simulink model "TrailerSoftware"  (R2019b)
settings: Solver=FixedStepDiscrete  StartTime=0.0  StopTime=inf  FixedStep=update  RelTol=1e-3  EnableMultiTasking=on
values from neighbouring files (symbols this model uses):
  countmax1 = 2500    [ProductionMfile.m]
  countmax2 = 2500    [ProductionMfile.m]
  HeaterIntGain = .0008    (= 0.0008)    [ProductionMfile.m]
  HeatGain = 10    [ProductionMfile.m]
  Intll = 0    [ProductionMfile.m]
  MaxCondPressure = 350    [ProductionMfile.m]
  MinSP = 1    [ProductionMfile.m]
  PostGain100 = 0.0002    [ProductionMfile.m]
  PostGain150 = 0.0005    [ProductionMfile.m]
  PostGain200 = 0.0004    [ProductionMfile.m]
  PostGain300 = 0.0008    [ProductionMfile.m]
  PostInit150 = 12    [ProductionMfile.m]
  PostIntulC = 65    [ProductionMfile.m]
  PostPGain = 0    [ProductionMfile.m]
  PreGain100 = 0.0005    [ProductionMfile.m]
  PreGain150 = 0.0005    [ProductionMfile.m]
  PreGain200 = 0.0003    [ProductionMfile.m]
  PreGain300 = 0.0008    [ProductionMfile.m]
  PreInit150 = 30    [ProductionMfile.m]
  PreIntulC = 65    [ProductionMfile.m]
  PreIntulDH = 65    [ProductionMfile.m]
  PrePGain = 0    [ProductionMfile.m]
  SatPress = [10 20 30 40 50 60 70 80 90 100 110 120 130 140 150 160 170      180 190 200 210 220 230 240 250 260 270 280 290 300 310 320 330      340 350 360 370 380 390 400 410 420 430 440 450 460 470 480 490      500]    [ProductionMfile.m]
  SatTemp = [-29.497 -2.4046 15.401 29.047 40.267 49.88 58.338 65.922 72.819      79.159 85.037 90.526 95.68 100.55 105.16 109.54 113.73 117.73 121.57      125.26 128.82 132.25 135.56 138.77 141.88 144.89 147.82 150.67 153.44      156.15 158.78 161.35 163.85 166.3 168.7 171.04 173.33 175.58 177.77      179.93 182.04 184.11 186.14 188.14 190.09 192.01 193.9 195.75 197.58      199.37]    [ProductionMfile.m]
  SHGain = 2    [ProductionMfile.m]
  SizeCANMatrix = 80    [ProductionMfile.m]
  SizeCOBIDVector = 10    [ProductionMfile.m]
  update = 0.002    [ProductionMfile.m]
undefined symbols (not defined in the file or in its folder): DiscIntNeverNeededParam, PostDGain, PreDGain, Ratio100, Ratio150, Ratio200, Ratio300
libraries: simulink x60, c2837xDlib x35, xpcutilitieslib x24, c2802xlib x8, c280xlib x7, etargetslib x4, svdutilitieslib x2, c2000lib x1
(part 3 of 8)

== system TrailerSoftware/Subsystem/Heating ==
  Heater Command Temp : Inport
  Duct Temp : Inport  Port=2
  UseHeater : Inport  Port=3
  Test Mode : Inport  Port=4
  BiPassHeatCom : Inport  Port=5
  PrePlusPost : Inport  Port=6
  Tamb : Inport  Port=7
  Tmode1 : Inport  Port=8
  Constant1 : Constant  Value=0
  Constant2 : Constant  Value=100
  Constant3 : Constant  Value=0
  Digital Clock : DigitalClock  SampleTime=update
  Discrete-Time Integrator : DiscreteIntegrator  SampleTime=-1  LimitOutput=on  UpperSaturationLimit=100  LowerSaturationLimit=0  ICPrevOutput=DiscIntNeverNeededParam  ICPrevScaledInput=DiscIntNeverNeededParam
  Gain1 : Gain  Gain=HeatGain
  Gain2 : Gain  Gain=HeaterIntGain
  MATLAB Function : MATLAB Function  Commented=on  TreatAsAtomicUnit=on
  Relational Operator : RelationalOperator  OutDataTypeStr=boolean  RndMeth=Simplest
  Saturation : Saturate  UpperLimit=100  LowerLimit=0
  Saturation1 : Saturate  UpperLimit=100  LowerLimit=0
  Saturation2 : Saturate  UpperLimit=10  LowerLimit=-10
  Sum : Sum  Inputs=|+-
  Sum1 : Sum  Inputs=|++
  Switch : Switch  Criteria=u2 ~= 0
  Switch1 : Switch  Criteria=u2 ~= 0
  Switch2 : Switch  Criteria=u2 ~= 0
  Heater Command : Outport  VectorParamsAs1DForOutWhenUnconnected=off
  Heater Error : Outport  Port=2  VectorParamsAs1DForOutWhenUnconnected=off
  wires:
  Gain1/1 -> Sum1/1  "%"
  Duct Temp/1 -> Sum/2
  Saturation/1 -> Switch/1
  UseHeater/1 -> Switch/2
  Constant1/1 -> Switch/3
  Test Mode/1 -> Switch2/2
  Switch/1 -> Switch2/3
  BiPassHeatCom/1 -> Switch2/1
  Switch2/1 -> Saturation1/1, MATLAB Function/2(In)
  Sum1/1 -> Relational Operator/1, Heater Error/1, Saturation/1
  Discrete-Time Integrator/1 -> Sum1/2
  Switch1/1 -> Discrete-Time Integrator/1
  Heater Command Temp/1 -> Sum/1
  Saturation1/1 -> Heater Command/1
  PrePlusPost/1 -> MATLAB Function/1(PrePlusPost)
  Tamb/1 -> MATLAB Function/3(Tamb)
  Digital Clock/1 -> MATLAB Function/4(time)
  Tmode1/1 -> MATLAB Function/5(tmode)
  Saturation2/1 -> Gain2/1
  Constant2/1 -> Relational Operator/2
  Sum/1 -> Gain1/1, Saturation2/1
  Gain2/1 -> Switch1/3
  Constant3/1 -> Switch1/1
  Relational Operator/1 -> Switch1/2

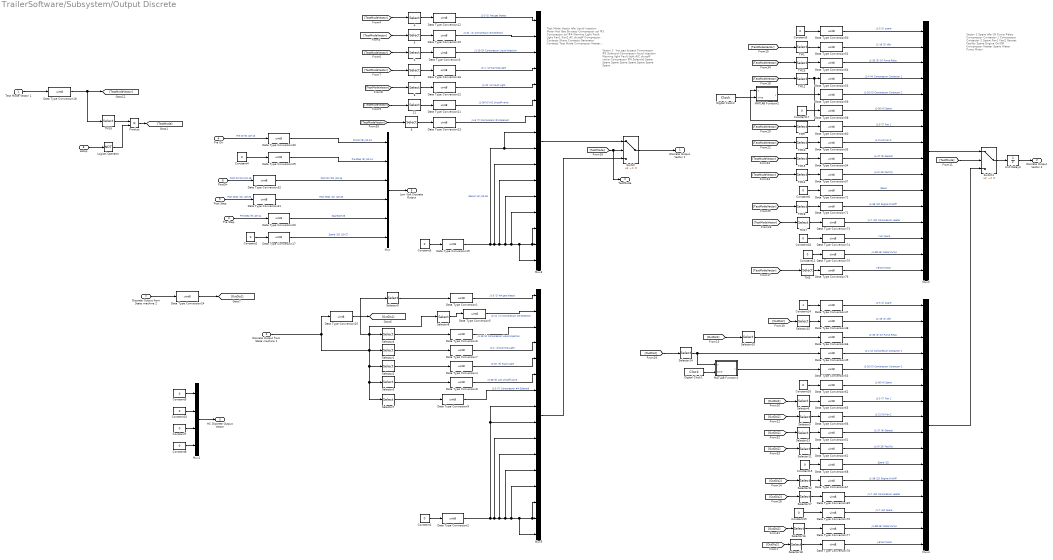
== system TrailerSoftware/Subsystem/Output Discrete ==
  note: Test Mode Vector
      | Idle
      | Liquid injection
      | Motor
      | Hot Gas By-pass
      | Compressor sol #3
      | Compressor sol #4
      | Warning Light
      | Fault Light
      | Fan1
      | Fan2
      | AC shutoff
      | Compressor Contacts
      |
      | Shore Contacts
      | Generator Contacts
      | Test Mode
      | Compressor Heater Contacts
      | Engine On/Off
      | Compressor Heater Contacts
      | Manual Operate Expan Valve
      | Init Expan valve
      | Reset Expan valve
      | Enable Expan valve
      | Oil Pump
  note: Vector 1`
      | hot gas bypass
      | Compressor #3 Solenoid
      | Compressor liquid injection
      | Warning light
      | Fault light
      | A/C shutoff valve
      | Compressor #4 Solenoid
      | Spare
      | Spare
      | Spare
      | Spare
      | Spare
      | Spare
      | Spare
      | Spare
  note: Vector 2
      | Spare
      | Idle
      | Oil Pump Relay
      | Compressor Contactor 1
      | Compressor Contactor 2
      | Spare
      | Fan1
      | Fan2
      | Genset
      | Facility
      | Spare
      | Engine On/Off
      | Compressor Heater
      | Spare
      | Water Pump
      | Motor
  Test Mode Vector 1 : Inport
  Discrete Output from State machine 1 : Inport  Port=2
  Pre Step : Inport  Port=3
  Pre Dir : Inport  Port=4
  Post Step : Inport  Port=5
  PostDir : Inport  Port=6
  Discrete Output from State machine 2 : Inport  Port=7
  estop : Inport  Port=8
  11 : Selector  InputPortWidth=ByPassVector  IndexOptions=Index vector (dialog)  Indices=[11]  OutputSizes=1
  2 : Selector  InputPortWidth=ByPassVector  IndexOptions=Index vector (dialog)  Indices=[2]  OutputSizes=1
  4 : Selector  InputPortWidth=ByPassVector  IndexOptions=Index vector (dialog)  Indices=[4]  OutputSizes=1
  5 : Selector  InputPortWidth=ByPassVector  IndexOptions=Index vector (dialog)  Indices=[5]  OutputSizes=1
  6 : Selector  InputPortWidth=ByPassVector  IndexOptions=Index vector (dialog)  Indices=[6]  OutputSizes=1
  7 : Selector  InputPortWidth=ByPassVector  IndexOptions=Index vector (dialog)  Indices=[7]  OutputSizes=1
  8 : Selector  InputPortWidth=ByPassVector  IndexOptions=Index vector (dialog)  Indices=[8]  OutputSizes=1
  Constant{1..6,11,15..19} (12 alike) : Constant  Value=0
  Constant{7..10} (4 alike) : Constant  Value=0  OutDataTypeStr=uint8
  Constant14 : Constant
  Data Type Conversion{1..9,12,15..25,29..32,47..78} (57 alike) : DataTypeConversion  OutDataTypeStr=uint8
  Digital Clock1 : DigitalClock  SampleTime=update
  Digital Clock2 : DigitalClock  SampleTime=update
  Logical Operator : Logic  Operator=NOT  AllPortsSameDT=off  OutDataTypeStr=boolean
  MATLAB Function1 : MATLAB Function  TreatAsAtomicUnit=on
  MATLAB Function2 : MATLAB Function  TreatAsAtomicUnit=on
  Mux : Mux  Inputs=6
  Mux1 : Mux
  Mux{2..5} (4 alike) : Mux  Inputs=16
  Product : Product
  Selector1 : Selector  InputPortWidth=16  IndexOptions=Index vector (dialog)  Indices=[4]  OutputSizes=1
  Selector10 : Selector  InputPortWidth=16  IndexOptions=Index vector (dialog)  Indices=[3]  OutputSizes=1
  Selector11 : Selector  InputPortWidth=16  IndexOptions=Index vector (dialog)  Indices=[10]  OutputSizes=1
  Selector12 : Selector  InputPortWidth=16  IndexOptions=Index vector (dialog)  Indices=[12]  OutputSizes=1
  Selector13 : Selector  InputPortWidth=16  IndexOptions=Index vector (dialog)  Indices=[9]  OutputSizes=1
  Selector14 : Selector  InputPortWidth=16  IndexOptions=Index vector (dialog)  Indices=[4]  OutputSizes=1
  Selector15 : Selector  InputPortWidth=16  IndexOptions=Index vector (dialog)  Indices=[2]  OutputSizes=1
  Selector16 : Selector  InputPortWidth=16  IndexOptions=Index vector (dialog)  Indices=[15]  OutputSizes=1
  Selector17 : Selector  InputPortWidth=16  IndexOptions=Index vector (dialog)  Indices=[13]  OutputSizes=1
  Selector18 : Selector  InputPortWidth=16  IndexOptions=Index vector (dialog)  Indices=[16]  OutputSizes=1
  Selector2 : Selector  InputPortWidth=16  IndexOptions=Index vector (dialog)  Indices=[8]  OutputSizes=1
  Selector3 : Selector  InputPortWidth=16  IndexOptions=Index vector (dialog)  Indices=[6]  OutputSizes=1
  Selector4 : Selector  InputPortWidth=16  IndexOptions=Index vector (dialog)  Indices=[3]  OutputSizes=1
  Selector5 : Selector  InputPortWidth=16  IndexOptions=Index vector (dialog)  Indices=[8]  OutputSizes=1
  Selector6 : Selector  InputPortWidth=16  IndexOptions=Index vector (dialog)  Indices=[7]  OutputSizes=1
  Selector7 : Selector  InputPortWidth=16  IndexOptions=Index vector (dialog)  Indices=[7]  OutputSizes=1
  Selector8 : Selector  InputPortWidth=16  IndexOptions=Index vector (dialog)  Indices=[2]  OutputSizes=1
  Selector9 : Selector  InputPortWidth=16  IndexOptions=Index vector (dialog)  Indices=[1]  OutputSizes=1
  Switch : Switch  Criteria=u2 ~= 0
  Switch1 : Switch  Criteria=u2 ~= 0
  TM1 : Selector  InputPortWidth=ByPassVector  IndexOptions=Index vector (dialog)  Indices=[1]  OutputSizes=1
  TM10 : Selector  InputPortWidth=ByPassVector  IndexOptions=Index vector (dialog)  Indices=[10]  OutputSizes=1
  TM12 : Selector  InputPortWidth=ByPassVector  IndexOptions=Index vector (dialog)  Indices=[12]  OutputSizes=1
  TM14 : Selector  InputPortWidth=ByPassVector  IndexOptions=Index vector (dialog)  Indices=[14]  OutputSizes=1
  "TM15 " : Selector  InputPortWidth=ByPassVector  IndexOptions=Index vector (dialog)  Indices=[15]  OutputSizes=1
  TM16 : Selector  InputPortWidth=ByPassVector  IndexOptions=Index vector (dialog)  Indices=[16]  OutputSizes=1
  TM17 : Selector  InputPortWidth=ByPassVector  IndexOptions=Index vector (dialog)  Indices=[17]  OutputSizes=1
  "TM18 " : Selector  InputPortWidth=ByPassVector  IndexOptions=Index vector (dialog)  Indices=[18]  OutputSizes=1
  TM23 : Selector  InputPortWidth=ByPassVector  IndexOptions=Index vector (dialog)  Indices=[23]  OutputSizes=1
  TM3 : Selector  InputPortWidth=ByPassVector  IndexOptions=Index vector (dialog)  Indices=[3]  OutputSizes=1
  TM9 : Selector  InputPortWidth=ByPassVector  IndexOptions=Index vector (dialog)  Indices=[9]  OutputSizes=1
  Unit Delay3 : UnitDelay  SampleTime=-1  HasFrameUpgradeWarning=on
  "Discrete Output Vector 1 " : Outport  OutDataTypeStr=uint8  PortDimensions=DiscreteOutputSize  SampleTime=update  VectorParamsAs1DForOutWhenUnconnected=off
  Discrete Output Vector 2 : Outport  Port=2  OutDataTypeStr=uint8  PortDimensions=16  SampleTime=update  VectorParamsAs1DForOutWhenUnconnected=off  LockScale=on
  "HC Discrete Output Vector " : Outport  Port=3  OutDataTypeStr=uint8  PortDimensions=HCDiscreteOutputSize  SampleTime=update  VectorParamsAs1DForOutWhenUnconnected=off  LockScale=on
  TestMode : Outport  Port=4  OutDataTypeStr=uint8  SampleTime=update  VectorParamsAs1DForOutWhenUnconnected=off
  Low Volt Discrete Output : Outport  Port=5  OutDataTypeStr=uint8  PortDimensions=SizeLowVoltDiscreteOutput  SampleTime=update  VectorParamsAs1DForOutWhenUnconnected=off
  wires:
  Test Mode Vector 1/1 -> Data Type Conversion18/1
  11/1 -> Data Type Conversion21/1
  Mux3/1 -> Switch/1
  7/1 -> Data Type Conversion16/1
  Data Type Conversion16/1 -> Mux3/4  "J1-4  (4)Warning Light"
  4/1 -> Data Type Conversion12/1
  Data Type Conversion12/1 -> Mux3/1  "J1-3 (1) hot gas bipass"
  5/1 -> Data Type Conversion15/1
  Data Type Conversion15/1 -> Mux3/2  "J1-21  (2) Compressor #3 Solenoid"
  Data Type Conversion3/1 -> Mux3/3  "J1-19 (3) Compressor Liquid Injection"
  Data Type Conversion21/1 -> Mux3/6  "J1-36 (6) A/C shutoff valve"
  [TestMode] -> TestMode/1, Switch/2
  8/1 -> Data Type Conversion22/1
  Data Type Conversion22/1 -> Mux3/5  "J1-20  (5) Fault Light"
  6/1 -> Data Type Conversion23/1
  Data Type Conversion1/1 -> Mux5/1  "J1-3 (1) hot gas bipass"
  Data Type Conversion6/1 -> Mux5/3  "J1-19 (3) Compressor Liquid Injection"
  Data Type Conversion7/1 -> Mux5/4  "J1-4  (4)Warning Light"
  Data Type Conversion4/1 -> Mux5/5  "J1-20  (5) Fault Light"
  Mux5/1 -> Switch/3
  Switch1/1 -> Unit Delay3/1
  Data Type Conversion30/1 -> Mux/1  "Pre Dir(8) J10-13"
  Data Type Conversion29/1 -> Mux/2  "Pre Step (9) J10-14"
  Data Type Conversion32/1 -> Mux/3  "Post Dir(10) J10-15"
  Switch/1 -> "Discrete Output Vector 1 "/1
  Data Type Conversion31/1 -> Mux/4  "Post Step (11) J10-25"
  Constant10/1 -> Mux1/2
  Constant9/1 -> Mux1/1
  Constant8/1 -> Mux1/4
  Constant7/1 -> Mux1/3
  Mux1/1 -> "HC Discrete Output Vector "/1
  Selector1/1 -> Data Type Conversion7/1
  Selector2/1 -> Data Type Conversion4/1
  Data Type Conversion8/1 -> Mux5/6  "J1-36 (6) A/C shutoff valve"
  Selector3/1 -> Data Type Conversion8/1
  Constant2/1 -> Data Type Conversion17/1
  Data Type Conversion17/1 -> Mux/6  "Spare (13) J10-27"
  Constant3/1 -> Data Type Conversion19/1
  Data Type Conversion19/1 -> Mux3/16, Mux3/15, Mux3/14, Mux3/13, Mux3/12, Mux3/11, Mux3/10, Mux3/8, Mux3/9  "Spare (14) J10-26"
  Data Type Conversion20/1 -> Mux/5  "SpareJ10-26"
  2/1 -> Data Type Conversion3/1
  [TestModeVector] -> 4/1
  [TestModeVector] -> 5/1
  [TestModeVector] -> 2/1
  [TestModeVector] -> 7/1
  [TestModeVector] -> 8/1
  [TestModeVector] -> 11/1
  Data Type Conversion64/1 -> Mux2/3  "J1-35 (3) Oil Pump Relay"
  Data Type Conversion60/1 -> Mux2/7  "J1-5 (7) Fan 1"
  Data Type Conversion58/1 -> Mux2/6  "J1-36 (6) Spare"
  Mux4/1 -> Switch1/3
  MATLAB Function2/1(y) -> Data Type Conversion59/1
  [TestMode] -> Switch1/2
  Data Type Conversion50/1 -> Mux2/1  "J1-3 (1) spare"
  Data Type Conversion53/1 -> Mux2/4  "J1-4 (4) Compressor Contactor 1"
  Data Type Conversion52/1 -> Mux2/2  "J1-19 (2) Idle"
  TM1/1 -> Data Type Conversion52/1
  Constant17/1 -> Data Type Conversion58/1
  Mux2/1 -> Switch1/1
  Data Type Conversion59/1 -> Mux2/5  "J1-20 (5) Compressor Contactor 2"
  [TestModeVector] -> TM1/1
  [TestModeVector] -> TM12/1
  TM9/1 -> Data Type Conversion60/1
  [TestModeVector] -> TM9/1
  [TestModeVector] -> TM10/1
  Data Type Conversion55/1 -> Mux2/8  "J1-21 (8) Fan 2"
  TM10/1 -> Data Type Conversion55/1
  Data Type Conversion54/1 -> Mux2/9  "J1-37 (9) Genset"
  [TestModeVector] -> "TM15 "/1
  "TM15 "/1 -> Data Type Conversion54/1
  Data Type Conversion57/1 -> Mux2/10  "J1-6 (10) Facility"
  TM14/1 -> Data Type Conversion57/1
  [TestModeVector] -> TM14/1
  [TestModeVector] -> "TM18 "/1
  "TM18 "/1 -> Data Type Conversion71/1
  Data Type Conversion71/1 -> Mux2/12  "J1-38 (12) Engine On/Off"
  Data Type Conversion72/1 -> Mux2/11  "Spare"
  Constant6/1 -> Data Type Conversion72/1
  TM17/1 -> Data Type Conversion73/1
  [TestModeVector] -> TM17/1
  Data Type Conversion73/1 -> Mux2/13  "J1-7 (13) Compressor Heater"
  Constant18/1 -> Data Type Conversion74/1
  Data Type Conversion74/1 -> Mux2/14  "(14) spare"
  Data Type Conversion75/1 -> Mux2/15  "J1-39(15) Water Pump"
  Data Type Conversion76/1 -> Mux2/16  "J-8(16) Motor"
  Data Type Conversion67/1 -> Mux4/12  "J1-38 (12) Engine On/Off"
  Data Type Conversion77/1 -> Mux4/15  "J1-39(15) Water Pump"
  Data Type Conversion56/1 -> Mux4/8  "J1-21 (8) Fan 2"
  Data Type Conversion78/1 -> Mux4/16  "J-8(16) Motor"
  Data Type Conversion68/1 -> Mux4/11  "Spare (11)"
  Data Type Conversion63/1 -> Mux4/5  "J1-20 (5) Compressor Contactor 2"
  Data Type Conversion49/1 -> Mux4/4  "J1-4 (4) Compressor Contactor 1"
  Data Type Conversion48/1 -> Mux4/2  "J1-19 (2) Idle"
  Data Type Conversion62/1 -> Mux4/6  "J1-36 (6) Spare"
  Data Type Conversion66/1 -> Mux4/3  "J1-35 (3) Oil Pump Relay"
  Data Type Conversion51/1 -> Mux4/9  "J1-37 (9) Genset"
  Data Type Conversion70/1 -> Mux4/14  "J1-7 (14) Spare"
  Data Type Conversion47/1 -> Mux4/1  "J1-3 (1) spare"
  Data Type Conversion65/1 -> Mux4/7  "J1-5 (7) Fan 1"
  Data Type Conversion61/1 -> Mux4/10  "J1-6 (10) Facility"
  Data Type Conversion69/1 -> Mux4/13  "J1-7 (13) Compressor Heater"
  Constant5/1 -> Data Type Conversion50/1
  Constant14/1 -> Data Type Conversion47/1
  Selector15/1 -> Data Type Conversion48/1
  [OutDis2] -> Selector6/1
  Selector6/1 -> Data Type Conversion65/1
  [OutDis2] -> Selector5/1
  Selector5/1 -> Data Type Conversion56/1
  Selector13/1 -> Data Type Conversion51/1
  Selector11/1 -> Data Type Conversion61/1
  Constant15/1 -> Data Type Conversion68/1
  Constant16/1 -> Data Type Conversion62/1
  MATLAB Function1/1(y) -> Data Type Conversion63/1
  Selector14/1 -> Data Type Conversion49/1, MATLAB Function1/1(u)
  [OutDis2] -> Selector12/1
  Selector12/1 -> Data Type Conversion67/1
  Digital Clock1/1 -> MATLAB Function1/2(time)
  [OutDis2] -> Selector14/1
  [OutDis2] -> Selector15/1
  Constant19/1 -> Data Type Conversion70/1
  [OutDis2] -> Selector16/1
  Selector16/1 -> Data Type Conversion77/1
  [TestModeVector] -> TM3/1
  [OutDis2] -> Selector17/1
  Selector17/1 -> Data Type Conversion69/1
  Selector4/1 -> Data Type Conversion6/1
  [OutDis2] -> Selector10/1
  Selector10/1 -> Data Type Conversion66/1
  [OutDis2] -> Selector13/1
  [OutDis2] -> Selector11/1
  Discrete Output from State machine 2/1 -> Data Type Conversion24/1
  Data Type Conversion18/1 -> TM16/1, [TestModeVector]
  Data Type Conversion24/1 -> [OutDis2]
  Data Type Conversion25/1 -> [OutDis1]
  Unit Delay3/1 -> Discrete Output Vector 2/1
  TM3/1 -> Data Type Conversion76/1
  [TestModeVector] -> TM23/1
  TM23/1 -> Data Type Conversion64/1
  [TestModeVector] -> 6/1
  Mux/1 -> Low Volt Discrete Output/1
  Post Step/1 -> Data Type Conversion31/1  "Post Step (11) J10-25"
  PostDir/1 -> Data Type Conversion32/1  "Post Dir(10) J10-15"
  Pre Step/1 -> Data Type Conversion20/1  "Pre Step (9) J10-14"
  Pre Dir/1 -> Data Type Conversion30/1  "Pre Dir(8) J10-13"
  Selector7/1 -> Data Type Conversion9/1
  Data Type Conversion9/1 -> Mux5/7  "J1-5 (7) Compressor #4 Solenoid"
  Data Type Conversion2/1 -> Mux5/8, Mux5/9, Mux5/10, Mux5/11, Mux5/12, Mux5/13, Mux5/16, Mux5/15, Mux5/14
  Constant1/1 -> Data Type Conversion2/1
  Constant4/1 -> Data Type Conversion29/1
  Digital Clock2/1 -> MATLAB Function2/2(time)
  TM12/1 -> MATLAB Function2/1(u), Data Type Conversion53/1
  Constant11/1 -> Data Type Conversion75/1
  Selector8/1 -> Data Type Conversion5/1
  Discrete Output from State machine 1/1 -> Selector8/1, Selector9/1, Selector4/1, Selector7/1, Selector3/1, Selector2/1, Selector1/1, Data Type Conversion25/1
  Data Type Conversion5/1 -> Mux5/2  "J1-21  (2) Compressor #3 Solenoid"
  Selector9/1 -> Data Type Conversion1/1
  Selector18/1 -> Data Type Conversion78/1
  Data Type Conversion23/1 -> Mux3/7  "J1-5 (7) Compressor #4 Solenoid"
  [OutDis2] -> Selector18/1
  estop/1 -> Logical Operator/1
  TM16/1 -> Product/1
  Product/1 -> [TestMode]
  Logical Operator/1 -> Product/2

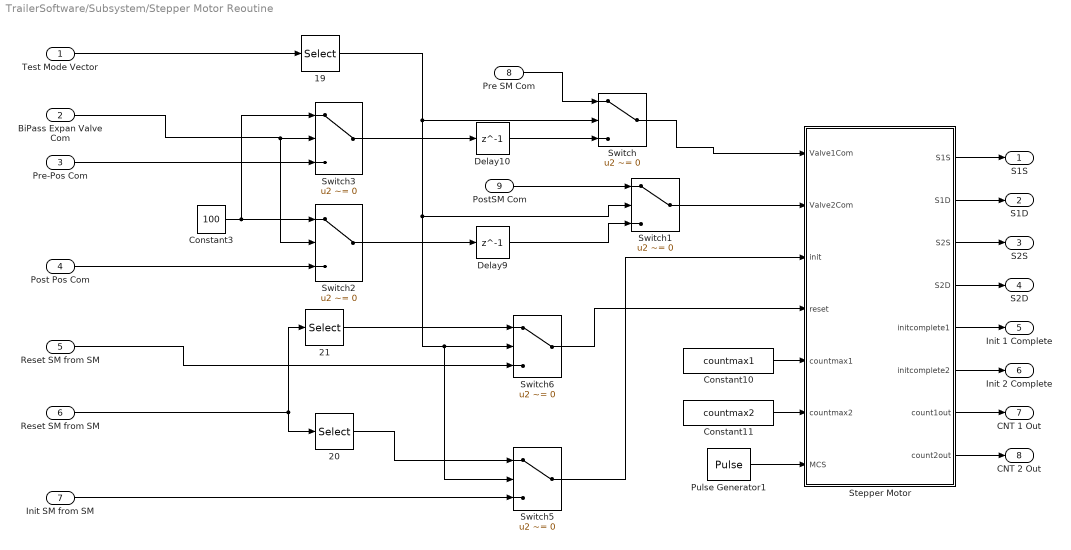
== system TrailerSoftware/Subsystem/Stepper Motor Reoutine ==
  Test Mode Vector : Inport
  BiPass Expan Valve Com : Inport  Port=2
  Pre-Pos Com : Inport  Port=3
  Post Pos Com : Inport  Port=4
  Reset SM from SM : Inport  Port=5
  Reset SM from SM : Inport  Port=6
  Init SM from SM : Inport  Port=7
  Pre SM Com : Inport  Port=8
  PostSM Com : Inport  Port=9
  "19 " : Selector  InputPortWidth=ByPassVector  IndexOptions=Index vector (dialog)  Indices=[19]  OutputSizes=1
  "20 " : Selector  InputPortWidth=ByPassVector  IndexOptions=Index vector (dialog)  Indices=[20]  OutputSizes=1
  21 : Selector  InputPortWidth=ByPassVector  IndexOptions=Index vector (dialog)  Indices=[21]  OutputSizes=1
  Constant10 : Constant  Value=countmax1
  Constant11 : Constant  Value=countmax2
  Constant3 : Constant  Value=100
  Delay10 : Delay  DelayLength=1  InitialCondition=0
  Delay9 : Delay  DelayLength=1  InitialCondition=0
  Pulse Generator1 : DiscretePulseGenerator  SampleTime=update
  "Stepper Motor " : MATLAB Function  TreatAsAtomicUnit=on
  Switch{,1..3,5..6} (6 alike) : Switch  Criteria=u2 ~= 0
  S1S : Outport
  S1D : Outport  Port=2
  S2S : Outport  Port=3
  S2D : Outport  Port=4
  Init 1 Complete : Outport  Port=5
  Init 2 Complete : Outport  Port=6
  CNT 1 Out : Outport  Port=7
  CNT 2 Out : Outport  Port=8
  wires:
  Constant10/1 -> "Stepper Motor "/5(countmax1)
  Constant3/1 -> Switch3/1, Switch2/1
  "19 "/1 -> Switch5/2, Switch6/2, Switch1/2, Switch/2
  PostSM Com/1 -> Switch1/1
  BiPass Expan Valve Com/1 -> Switch3/2, Switch2/2
  "Stepper Motor "/3(S2S) -> S2S/1
  "Stepper Motor "/6(initcomplete2) -> Init 2 Complete/1
  Switch6/1 -> "Stepper Motor "/4(reset)
  Switch1/1 -> "Stepper Motor "/2(Valve2Com)
  Pre-Pos Com/1 -> Switch3/3
  Reset SM from SM/1 -> "20 "/1, 21/1
  "20 "/1 -> Switch5/1
  Switch5/1 -> "Stepper Motor "/3(init)
  Switch2/1 -> Delay9/1
  Pulse Generator1/1 -> "Stepper Motor "/7(MCS)
  Test Mode Vector/1 -> "19 "/1
  Delay10/1 -> Switch/3
  Constant11/1 -> "Stepper Motor "/6(countmax2)
  Switch3/1 -> Delay10/1
  Post Pos Com/1 -> Switch2/3
  Delay9/1 -> Switch1/3
  21/1 -> Switch6/1
  Switch/1 -> "Stepper Motor "/1(Valve1Com)
  "Stepper Motor "/5(initcomplete1) -> Init 1 Complete/1
  "Stepper Motor "/4(S2D) -> S2D/1
  "Stepper Motor "/7(count1out) -> CNT 1 Out/1
  Reset SM from SM/1 -> Switch6/3
  "Stepper Motor "/1(S1S) -> S1S/1
  Init SM from SM/1 -> Switch5/3
  "Stepper Motor "/2(S1D) -> S1D/1
  "Stepper Motor "/8(count2out) -> CNT 2 Out/1
  Pre SM Com/1 -> Switch/1

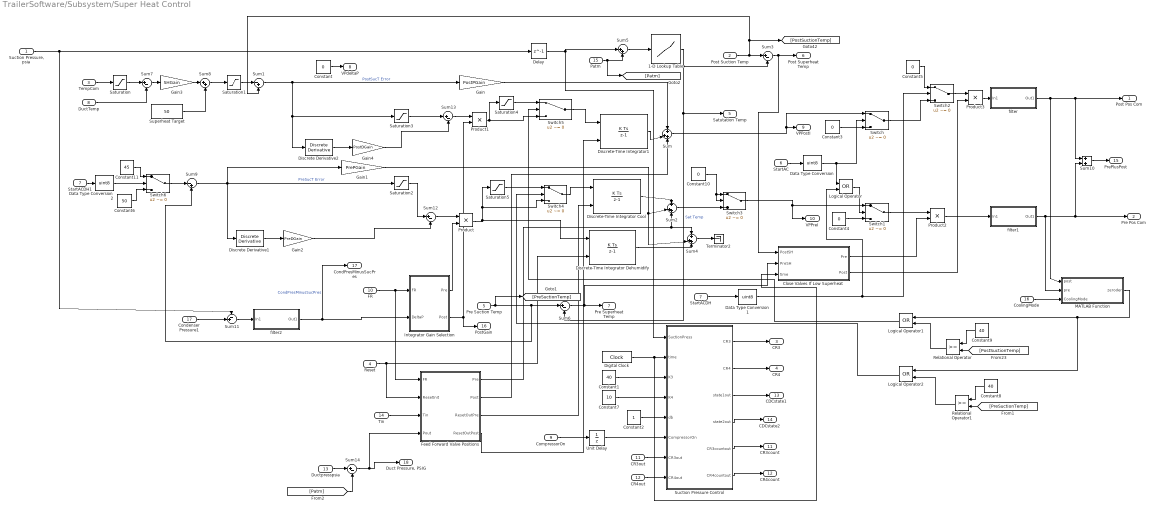
== system TrailerSoftware/Subsystem/Super Heat Control ==
  "Suction Pressure, psia" : Inport
  Post Suction Temp : Inport  Port=2
  TempCom : Inport  Port=3
  Reset : Inport  Port=4
  Pre Suction Temp : Inport  Port=5
  StartAC : Inport  Port=6
  StartACDH : Inport  Port=7
  DuctTemp : Inport  Port=8
  CompressorOn : Inport  Port=9
  FR : Inport  Port=10
  CR3out : Inport  Port=11
  CR4out : Inport  Port=12
  Ductpresspsia : Inport  Port=13
  Tin : Inport  Port=14
  Patm : Inport  Port=15
  CoolingMode : Inport  Port=16
  Condenser Pressure1 : Inport  Port=17
  1-D Lookup Table : Lookup_n-D  NumberOfTableDimensions=1  BreakpointsForDimension1=SatPress  Table=SatTemp  InternalRulePriority=Speed  RndMeth=Simplest  InputSameDT=on
  Close Valves If Low Superheat : MATLAB Function  TreatAsAtomicUnit=on
  Constant{,3..5,10} (5 alike) : Constant  Value=0
  Constant1 : Constant  Value=40
  Constant11 : Constant  Value=45
  Constant2 : Constant
  Constant6 : Constant  Value=50
  Constant7 : Constant  Value=10
  Constant8 : Constant  Value=40
  Constant9 : Constant  Value=40
  Data Type Conversion : DataTypeConversion  OutDataTypeStr=uint8
  Data Type Conversion1 : DataTypeConversion  OutDataTypeStr=uint8
  Data Type Conversion2 : DataTypeConversion  OutDataTypeStr=uint8
  Delay : Delay  DelayLength=1  InitialCondition=0
  Digital Clock : DigitalClock  SampleTime=update
  Discrete Derivative1 : simulink/Discrete/Discrete Derivative  gainval=1.0  ICPrevScaledInput=0.0  OutMin=[]  OutMax=[]  OutDataType=fixdt(1, 16)  OutScaling=2^-10  DoSatur=on
  Discrete Derivative2 : simulink/Discrete/Discrete Derivative  gainval=1.0  ICPrevScaledInput=0.0  OutMin=[]  OutMax=[]  OutDataType=fixdt(1, 16)  OutScaling=2^-10  DoSatur=on
  Discrete-Time Integrator Cool : DiscreteIntegrator  ExternalReset=level  SampleTime=-1  LimitOutput=on  UpperSaturationLimit=PreIntulC  LowerSaturationLimit=Intll  ICPrevOutput=DiscIntNeverNeededParam  ICPrevScaledInput=DiscIntNeverNeededParam
  Discrete-Time Integrator Dehumidify : DiscreteIntegrator  ExternalReset=level  SampleTime=-1  LimitOutput=on  UpperSaturationLimit=PreIntulDH  LowerSaturationLimit=Intll  ICPrevOutput=DiscIntNeverNeededParam  ICPrevScaledInput=DiscIntNeverNeededParam
  Discrete-Time Integrator1 : DiscreteIntegrator  ExternalReset=level  SampleTime=-1  LimitOutput=on  UpperSaturationLimit=PostIntulC  LowerSaturationLimit=Intll  ICPrevOutput=DiscIntNeverNeededParam  ICPrevScaledInput=DiscIntNeverNeededParam
  Feed Forward Valve Positions : MATLAB Function  TreatAsAtomicUnit=on
  Gain : Gain  Gain=PostPGain
  Gain1 : Gain  Gain=PrePGain
  Gain2 : Gain  Gain=PreDGain
  Gain3 : Gain  Gain=SHGain
  Gain4 : Gain  Gain=PostDGain
  Integrator Gain Selection : MATLAB Function  TreatAsAtomicUnit=on
  Logical Operator : Logic  Operator=OR  AllPortsSameDT=off  OutDataTypeStr=boolean
  Logical Operator1 : Logic  Operator=OR  AllPortsSameDT=off  OutDataTypeStr=boolean
  Logical Operator2 : Logic  Operator=OR  AllPortsSameDT=off  OutDataTypeStr=boolean
  MATLAB Function : MATLAB Function  TreatAsAtomicUnit=on
  Product{,1..3} (4 alike) : Product
  Relational Operator : RelationalOperator  OutDataTypeStr=boolean  RndMeth=Simplest
  Relational Operator1 : RelationalOperator  OutDataTypeStr=boolean  RndMeth=Simplest
  Saturation : Saturate  UpperLimit=80  LowerLimit=45
  Saturation1 : Saturate  UpperLimit=80  LowerLimit=40
  Saturation2 : Saturate  UpperLimit=10  LowerLimit=-10
  Saturation3 : Saturate  UpperLimit=10  LowerLimit=-10
  Saturation4 : Saturate  UpperLimit=0  LowerLimit=-10
  Saturation5 : Saturate  UpperLimit=0  LowerLimit=-10
  StartACDH1 : InportShadow  Port=7
  Suction Pressure Control : MATLAB Function  TreatAsAtomicUnit=on
  Sum : Sum  Inputs=+|++
  Sum1 : Sum  Inputs=|-+
  Sum10 : Sum
  Sum11 : Sum  Inputs=-+|
  Sum{3,6..7,12..14} (6 alike) : Sum  Inputs=|+-
  Sum2 : Sum  Inputs=+|++
  Sum4 : Sum  Inputs=+|++
  Sum5 : Sum  Inputs=|++
  Sum8 : Sum  Inputs=|++
  Sum9 : Sum  Inputs=|-+
  Superheat Target : Constant  Value=50
  Switch{,1..6} (7 alike) : Switch  Criteria=u2 ~= 0
  Terminator2 : Terminator
  Unit Delay : UnitDelay  SampleTime=-1  HasFrameUpgradeWarning=on
  filter : Subsystem
  filter1 : Subsystem
  filter2 : Subsystem  Tag=CondPresMinusSucPres
  Post Pos Com : Outport  VectorParamsAs1DForOutWhenUnconnected=off
  Pre Pos Com : Outport  Port=2  VectorParamsAs1DForOutWhenUnconnected=off
  CR3 : Outport  Port=3  VectorParamsAs1DForOutWhenUnconnected=off
  CR4 : Outport  Port=4  VectorParamsAs1DForOutWhenUnconnected=off
  Satutation Temp : Outport  Port=5  VectorParamsAs1DForOutWhenUnconnected=off
  Post Superheat Temp : Outport  Port=6  VectorParamsAs1DForOutWhenUnconnected=off
  Pre Superheat Temp : Outport  Port=7  VectorParamsAs1DForOutWhenUnconnected=off
  VPdeltaP : Outport  Port=8  VectorParamsAs1DForOutWhenUnconnected=off
  VPPostI : Outport  Port=9  VectorParamsAs1DForOutWhenUnconnected=off
  VPPreI : Outport  Port=10  VectorParamsAs1DForOutWhenUnconnected=off
  CR3count : Outport  Port=11  VectorParamsAs1DForOutWhenUnconnected=off
  CR4count : Outport  Port=12  VectorParamsAs1DForOutWhenUnconnected=off
  CDCstate1 : Outport  Port=13  VectorParamsAs1DForOutWhenUnconnected=off
  CDCstate2 : Outport  Port=14  VectorParamsAs1DForOutWhenUnconnected=off
  PrePlusPost : Outport  Port=15  VectorParamsAs1DForOutWhenUnconnected=off
  PostGain : Outport  Port=16  VectorParamsAs1DForOutWhenUnconnected=off
  CondPresMinusSucPres : Outport  Port=17  VectorParamsAs1DForOutWhenUnconnected=off
  "Duct Pressure, PSIG" : Outport  Port=18  VectorParamsAs1DForOutWhenUnconnected=off
  wires:
  Post Suction Temp/1 -> [PostSuctionTemp], Sum1/2, Sum3/1
  "Suction Pressure, psia"/1 -> Sum11/1, Delay/1
  Sum1/1 -> Gain/1, Saturation3/1, Discrete Derivative2/1  "PostSucT Error"
  Product1/1 -> Saturation4/1, Switch5/3
  1-D Lookup Table/1 -> Sum6/2, Satutation Temp/1, Sum3/2  "Sat Temp"
  Sum3/1 -> Close Valves If Low Superheat/1(PostSH), Post Superheat Temp/1
  Reset/1 -> Discrete-Time Integrator Dehumidify/2, Feed Forward Valve Positions/2(ResetInit)
  Constant/1 -> VPdeltaP/1
  Pre Suction Temp/1 -> Sum9/2, Sum6/1, [PreSuctionTemp]
  Sum6/1 -> Close Valves If Low Superheat/2(PreSH), Pre Superheat Temp/1
  Suction Pressure Control/3(state1out) -> CDCstate1/1
  Digital Clock/1 -> Close Valves If Low Superheat/3(time), Suction Pressure Control/2(time)
  Constant1/1 -> Suction Pressure Control/3(K3)
  Constant2/1 -> Suction Pressure Control/5(db)
  Suction Pressure Control/1(CR3) -> CR3/1
  Suction Pressure Control/2(CR4) -> CR4/1
  Constant3/1 -> Switch/3
  Sum/1 -> Switch/1, VPPostI/1
  Switch3/1 -> VPPreI/1, Switch1/1
  Constant4/1 -> Switch1/3
  Switch/1 -> Switch2/3
  StartACDH/1 -> Data Type Conversion1/1
  Constant5/1 -> Switch2/1
  StartAC/1 -> Data Type Conversion/1
  Data Type Conversion/1 -> Logical Operator/1, Switch/2
  TempCom/1 -> Saturation/1
  Saturation/1 -> Sum7/1
  DuctTemp/1 -> Sum7/2
  Sum7/1 -> Gain3/1
  Saturation1/1 -> Sum1/1
  Sum8/1 -> Saturation1/1
  Superheat Target/1 -> Sum8/2
  Gain3/1 -> Sum8/1
  Data Type Conversion1/1 -> Logical Operator/2, Switch2/2
  Sum9/1 -> Gain1/1, Saturation2/1, Discrete Derivative1/1  "PreSucT Error"
  Suction Pressure Control/5(CR3countout) -> CR3count/1
  Suction Pressure Control/6(CR4countout) -> CR4count/1
  CompressorOn/1 -> Unit Delay/1
  Unit Delay/1 -> Suction Pressure Control/6(CompressorOn)
  Suction Pressure Control/4(state2out) -> CDCstate2/1
  FR/1 -> Feed Forward Valve Positions/1(FR), Integrator Gain Selection/1(FR)
  Integrator Gain Selection/2(Post) -> PostGain/1, Product1/2
  Integrator Gain Selection/1(Pre) -> Product/2
  Feed Forward Valve Positions/1(Pre) -> Sum4/1, Sum2/3
  Feed Forward Valve Positions/2(Post) -> Sum/3
  CR3out/1 -> Suction Pressure Control/7(CR3out)
  CR4out/1 -> Suction Pressure Control/8(CR4out)
  Discrete-Time Integrator Cool/1 -> Sum2/1
  Switch1/1 -> Product2/1
  Product2/1 -> filter1/1(In1)
  Close Valves If Low Superheat/1(Pre) -> Product2/2
  Switch2/1 -> Product3/1
  Close Valves If Low Superheat/2(Post) -> Product3/2
  Feed Forward Valve Positions/3(ResetOutPre) -> Discrete-Time Integrator Cool/2
  Feed Forward Valve Positions/4(ResetOutPost) -> Discrete-Time Integrator1/2
  Product3/1 -> filter/1(In1)
  Constant7/1 -> Suction Pressure Control/4(K4)
  Discrete-Time Integrator1/1 -> Sum/2
  Sum2/1 -> Switch3/3
  Tin/1 -> Feed Forward Valve Positions/3(Tin)
  Patm/1 -> [Patm], Sum5/2
  Sum5/1 -> 1-D Lookup Table/1
  Delay/1 -> Suction Pressure Control/1(SuctionPress), Sum5/1
  Gain/1 -> Sum/1
  Gain1/1 -> Sum4/2, Sum2/2
  Logical Operator/1 -> Switch1/2
  filter/1(Out1) -> MATLAB Function/1(post), Sum10/1, Post Pos Com/1
  filter1/1(Out1) -> Pre Pos Com/1, Sum10/2, MATLAB Function/2(pre)
  Product/1 -> Discrete-Time Integrator Dehumidify/1, Saturation5/1, Switch4/3
  Logical Operator1/1 -> Switch5/2
  Saturation4/1 -> Switch5/1
  Sum10/1 -> PrePlusPost/1
  CoolingMode/1 -> MATLAB Function/3(CoolingMode)
  MATLAB Function/1(zeroder) -> Logical Operator2/1, Logical Operator1/1
  Relational Operator/1 -> Logical Operator1/2
  Constant9/1 -> Relational Operator/1
  [PostSuctionTemp] -> Relational Operator/2
  [PreSuctionTemp] -> Relational Operator1/2
  Constant8/1 -> Relational Operator1/1
  Relational Operator1/1 -> Logical Operator2/2
  Saturation5/1 -> Switch4/1
  Logical Operator2/1 -> Switch4/2
  Constant10/1 -> Switch3/2, Switch3/1
  Sum4/1 -> Terminator2/1
  Discrete-Time Integrator Dehumidify/1 -> Sum4/3
  Switch4/1 -> Discrete-Time Integrator Cool/1
  Condenser Pressure1/1 -> Sum11/2
  Sum11/1 -> filter2/1(In1)
  filter2/1(Out1) -> CondPresMinusSucPres/1, Integrator Gain Selection/2(DeltaP)  "CondPresMinusSucPres"
  Switch5/1 -> Discrete-Time Integrator1/1
  Switch6/1 -> Sum9/1
  Constant11/1 -> Switch6/1
  StartACDH1/1 -> Data Type Conversion2/1
  Constant6/1 -> Switch6/3
  Data Type Conversion2/1 -> Switch6/2
  Discrete Derivative1/1 -> Gain2/1
  Gain2/1 -> Sum12/2
  Gain4/1 -> Sum13/2
  Discrete Derivative2/1 -> Gain4/1
  Sum12/1 -> Product/1
  Saturation2/1 -> Sum12/1
  Sum13/1 -> Product1/1
  Saturation3/1 -> Sum13/1
  Sum14/1 -> Feed Forward Valve Positions/4(Pout), "Duct Pressure, PSIG"/1
  Ductpresspsia/1 -> Sum14/1
  [Patm] -> Sum14/2

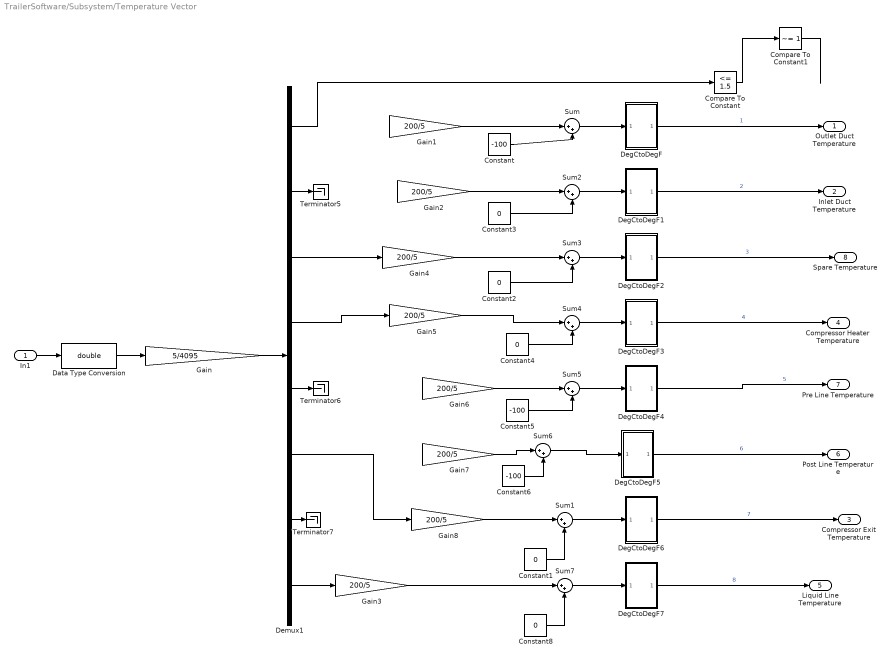
== system TrailerSoftware/Subsystem/Temperature Vector ==
  In1 : Inport
  Compare To Constant : simulink/Logic and Bit Operations/Compare To Constant  relop=<=  const=1.5  OutDataTypeStr=uint8
  Compare To Constant1 : simulink/Logic and Bit Operations/Compare To Constant  Description=Flipping the logic of the prior block, DB, 7/16/19  relop=~=  const=1  OutDataTypeStr=uint8
  Constant : Constant  Value=-100
  Constant{1..4,8} (5 alike) : Constant  Value=0
  Constant5 : Constant  Value=-100
  Constant6 : Constant  Value=-100
  Data Type Conversion : DataTypeConversion  OutDataTypeStr=double
  DegCtoDegF : Subsystem
  DegCtoDegF1 : Subsystem
  DegCtoDegF2 : Subsystem
  DegCtoDegF3 : Subsystem
  DegCtoDegF4 : Subsystem
  DegCtoDegF5 : Subsystem
  DegCtoDegF6 : Subsystem
  DegCtoDegF7 : Subsystem
  Demux1 : Demux  Outputs=8
  Gain : Gain  Gain=5/4095  OutDataTypeStr=double
  Gain{1..8} (8 alike) : Gain  Gain=200/5
  Sum{,1..7} (8 alike) : Sum  Inputs=|++
  Terminator5 : Terminator
  Terminator6 : Terminator
  Terminator7 : Terminator
  Outlet Duct Temperature : Outport  VectorParamsAs1DForOutWhenUnconnected=off
  Inlet Duct Temperature : Outport  Port=2  VectorParamsAs1DForOutWhenUnconnected=off
  Compressor Exit Temperature : Outport  Port=3  VectorParamsAs1DForOutWhenUnconnected=off
  Compressor Heater Temperature : Outport  Port=4  VectorParamsAs1DForOutWhenUnconnected=off
  Liquid Line Temperature : Outport  Port=5  VectorParamsAs1DForOutWhenUnconnected=off
  Post Line Temperature : Outport  Port=6  VectorParamsAs1DForOutWhenUnconnected=off
  Pre Line Temperature : Outport  Port=7  VectorParamsAs1DForOutWhenUnconnected=off
  Spare Temperature : Outport  Port=8  VectorParamsAs1DForOutWhenUnconnected=off
  wires:
  In1/1 -> Data Type Conversion/1
  Demux1/2 -> Terminator5/1
  Demux1/3 -> Gain4/1
  Demux1/4 -> Gain5/1
  Demux1/5 -> Terminator6/1
  Demux1/6 -> Gain8/1
  Demux1/8 -> Gain3/1
  Demux1/7 -> Terminator7/1
  Gain1/1 -> Sum/1
  Constant/1 -> Sum/2
  Sum2/1 -> DegCtoDegF1/1(In1)
  Gain3/1 -> Sum7/1
  Sum3/1 -> DegCtoDegF2/1(In1)
  Sum4/1 -> DegCtoDegF3/1(In1)
  Sum5/1 -> DegCtoDegF4/1(In1)
  Sum6/1 -> DegCtoDegF5/1(In1)
  Constant1/1 -> Sum1/2
  Gain8/1 -> Sum1/1
  Sum1/1 -> DegCtoDegF6/1(In1)
  Constant2/1 -> Sum3/2
  Constant3/1 -> Sum2/2
  Gain2/1 -> Sum2/1
  Gain4/1 -> Sum3/1
  Constant4/1 -> Sum4/2
  Gain5/1 -> Sum4/1
  Constant5/1 -> Sum5/2
  Gain6/1 -> Sum5/1
  Gain7/1 -> Sum6/1
  Constant6/1 -> Sum6/2
  Data Type Conversion/1 -> Gain/1
  DegCtoDegF3/1(Out1) -> Compressor Heater Temperature/1  "4"
  DegCtoDegF4/1(Out1) -> Pre Line Temperature/1  "5"
  DegCtoDegF5/1(Out1) -> Post Line Temperature/1  "6"
  DegCtoDegF1/1(Out1) -> Inlet Duct Temperature/1  "2"
  DegCtoDegF/1(Out1) -> Outlet Duct Temperature/1  "1"
  DegCtoDegF7/1(Out1) -> Liquid Line Temperature/1  "8"
  Constant8/1 -> Sum7/2
  Sum7/1 -> DegCtoDegF7/1(In1)
  Sum/1 -> DegCtoDegF/1(In1)
  Gain/1 -> Demux1/1
  DegCtoDegF2/1(Out1) -> Spare Temperature/1  "3"
  Demux1/1 -> Compare To Constant/1
  Compare To Constant/1 -> Compare To Constant1/1
  DegCtoDegF6/1(Out1) -> Compressor Exit Temperature/1  "7"
  Compare To Constant1/1 -> ?
